simulink model "NN1"  (R2016a)
settings: Solver=VariableStepAuto  StartTime=0.0  StopTime=10.0  RelTol=1e-3
values from neighbouring files (symbols this model uses):
  AaLinear = [0,1,0,0; -(K)/Md,-Rmd/Md,0,A/Md; 0,0,0,1; 0,-A/(L0+Ld),-(1/Cd)/(L0+Ld),-(Re0+Red)/(L0+Ld)]    [NeuroControl_loudspeaker.m]    (also in NeuroControl_loudspeaker2.m; NeuroControl_loudspeaker_LinearPlusNN.m; NeuroControl_loudspeaker_MoreLikeMachineLearning.m; NeuroControl_loudspeaker_MoreLikeMachineLearning_deep.m)
  Anlr = zeros(4,4)    [NeuroControl_loudspeaker.m]    (also in NeuroControl_loudspeaker2.m; NeuroControl_loudspeaker_LinearPlusNN.m; NeuroControl_loudspeaker_MoreLikeMachineLearning.m; NeuroControl_loudspeaker_MoreLikeMachineLearning_deep.m)
  Anlr2 = zeros(4,4)    [NeuroControl_loudspeaker.m]    (also in NeuroControl_loudspeaker2.m; NeuroControl_loudspeaker_LinearPlusNN.m; NeuroControl_loudspeaker_MoreLikeMachineLearning.m; NeuroControl_loudspeaker_MoreLikeMachineLearning_deep.m)
  Anlr3 = zeros(4,4)    [NeuroControl_loudspeaker.m]    (also in NeuroControl_loudspeaker2.m; NeuroControl_loudspeaker_LinearPlusNN.m; NeuroControl_loudspeaker_MoreLikeMachineLearning.m; NeuroControl_loudspeaker_MoreLikeMachineLearning_deep.m)
  Atemp = A    (= 5.62)    [NeuroControl_loudspeaker.m]    (also in NeuroControl_loudspeaker2.m; NeuroControl_loudspeaker_LinearPlusNN.m; NeuroControl_loudspeaker_MoreLikeMachineLearning.m; NeuroControl_loudspeaker_MoreLikeMachineLearning_deep.m)
  Ba = [0,0,0,1/(L0+Ld)]'    [NeuroControl_loudspeaker.m]    (also in NeuroControl_loudspeaker2.m; NeuroControl_loudspeaker_LinearPlusNN.m; NeuroControl_loudspeaker_MoreLikeMachineLearning.m; NeuroControl_loudspeaker_MoreLikeMachineLearning_deep.m)
  K = Kd    (= 4538)    [NeuroControl_loudspeaker.m]    (also in NeuroControl_loudspeaker2.m; NeuroControl_loudspeaker_LinearPlusNN.m; NeuroControl_loudspeaker_MoreLikeMachineLearning.m; NeuroControl_loudspeaker_MoreLikeMachineLearning_deep.m)
  noise = 0    [NeuroControl_loudspeaker.m]    (also in NeuroControl_loudspeaker2.m; NeuroControl_loudspeaker_LinearPlusNN.m; NeuroControl_loudspeaker_MoreLikeMachineLearning.m; NeuroControl_loudspeaker_MoreLikeMachineLearning_deep.m)
  plantInputGainCompensationFb = 1/1.15    (= 0.869565217391)    [NeuroControl_loudspeaker.m]    (also in NeuroControl_loudspeaker2.m; NeuroControl_loudspeaker_LinearPlusNN.m; NeuroControl_loudspeaker_MoreLikeMachineLearning.m; NeuroControl_loudspeaker_MoreLikeMachineLearning_deep.m)
  Rmd = 2.34    [NeuroControl_loudspeaker.m]    (also in NeuroControl_loudspeaker2.m; NeuroControl_loudspeaker_LinearPlusNN.m; NeuroControl_loudspeaker_MoreLikeMachineLearning.m; NeuroControl_loudspeaker_MoreLikeMachineLearning_deep.m)
settings Model: Creator=kadowaki  LastModifiedBy=kadowaki

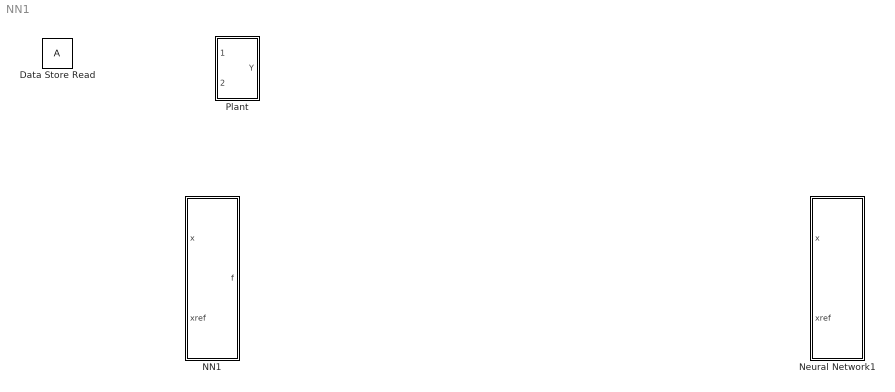
== system NN1 ==
  Data Store Read : DataStoreRead
  NN1 : MATLAB Function  TreatAsAtomicUnit=on
      settings: MinAlgLoopOccurrences=on
  Neural Network1 : MATLAB Function  TreatAsAtomicUnit=on
      settings: MinAlgLoopOccurrences=on
  Plant : Subsystem

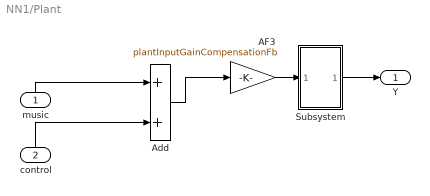
== system NN1/Plant ==
  music : Inport
  control : Inport  Port=2
  AF3 : Gain  Gain=plantInputGainCompensationFb
  Add : Sum
  Subsystem : Subsystem  TreatAsAtomicUnit=on
      settings: MinAlgLoopOccurrences=on
  Y : Outport
  wires:
  Subsystem/1(Out1) -> Y/1
  AF3/1 -> Subsystem/1(In2)
  music/1 -> Add/1
  control/1 -> Add/2
  Add/1 -> AF3/1

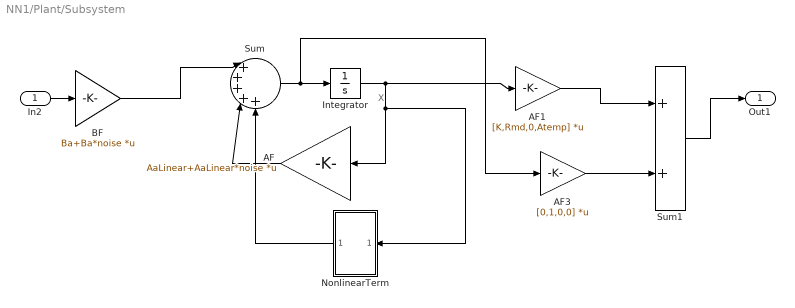
== system NN1/Plant/Subsystem ==
  note: X
  In2 : Inport
  AF : Gain  Gain=AaLinear+AaLinear*noise  Multiplication=Matrix(K*u)
  AF1 : Gain  Gain=[K,Rmd,0,Atemp]  Multiplication=Matrix(K*u)
  AF3 : Gain  Gain=[0,1,0,0]  Multiplication=Matrix(K*u)
  BF : Gain  Gain=Ba+Ba*noise  Multiplication=Matrix(K*u)
  Integrator : Integrator
  NonlinearTerm : Subsystem
  Sum : Sum  Inputs=|+++++
  Sum1 : Sum
  Out1 : Outport
  wires:
  BF/1 -> Sum/1
  Sum/1 -> Integrator/1, AF3/1
  Integrator/1 -> AF/1, NonlinearTerm/1(In1), AF1/1
  AF/1 -> Sum/4
  NonlinearTerm/1(Out2) -> Sum/5
  In2/1 -> BF/1
  AF1/1 -> Sum1/1
  Sum1/1 -> Out1/1
  AF3/1 -> Sum1/2

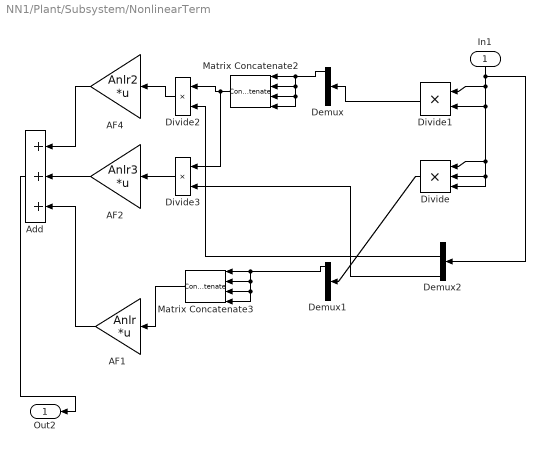
== system NN1/Plant/Subsystem/NonlinearTerm ==
  In1 : Inport
  AF1 : Gain  Gain=Anlr  Multiplication=Matrix(K*u)
  AF2 : Gain  Gain=Anlr3  Multiplication=Matrix(K*u)
  AF4 : Gain  Gain=Anlr2  Multiplication=Matrix(K*u)
  Add : Sum  Inputs=+++
  Demux : Demux  Outputs=[1,1,1,1]
  Demux1 : Demux  Outputs=[1,1,1,1]
  Demux2 : Demux  Outputs=[1,1,1,1]
  Divide : Product  Inputs=***
  Divide1 : Product  Inputs=**
  Divide2 : Product  Inputs=**
  Divide3 : Product  Inputs=**
  Matrix Concatenate2 : Concatenate  NumInputs=4
  Matrix Concatenate3 : Concatenate  NumInputs=4
  Out2 : Outport
  wires:
  Matrix Concatenate3/1 -> AF1/1
  Divide/1 -> Demux1/1
  In1/1 -> Demux2/1, Divide1/2, Divide/2, Divide/3, Divide/1, Divide1/1
  Demux/1 -> Matrix Concatenate2/1, Matrix Concatenate2/2, Matrix Concatenate2/3, Matrix Concatenate2/4
  Demux1/1 -> Matrix Concatenate3/1, Matrix Concatenate3/2, Matrix Concatenate3/3, Matrix Concatenate3/4
  AF2/1 -> Add/2
  AF4/1 -> Add/1
  AF1/1 -> Add/3
  Add/1 -> Out2/1
  Matrix Concatenate2/1 -> Divide2/1, Divide3/1
  Demux2/2 -> Divide2/2
  Divide2/1 -> AF4/1
  Divide3/1 -> AF2/1
  Demux2/4 -> Divide3/2
  Divide1/1 -> Demux/1

== matlab function NN1/Neural Network1 ==
  data: x input; xref input; yOld data_store_memory; duOld data_store_memory
function fcn(x,xref)
%% cost関数をatctual plantの出力YとYrefの差の二乗和の形に書き換える。それにともなってsigKとかも変わる
%%%%%%%%%%%%%%%%%%%%%%%%%%%%%%%%%%%%%%%%%%%%%%%%%%%%%%%%%%%%%%%%%%%%%%%%%%%%%%%%%%%%%%%%%%%%%%%%%%%%%%%%%%%%
%%

%#codegen
%配列は縦で入れる
%PRMLの5.3.2
%隠れ層はtanh,出力層は線形の活性化関数
% Input:
%   x: state vector of a plant
%   xref: reference state vector
%   h: 隠れ層のニューロン数
% Ouput:
%   du: input to compensate plant nonlinearity
%   mse: mean square error
%12input-1outputのニューラルネット
%フィードバックの機構いる？ニューラルネットだけではだめなのか。
%実装に際しては，1サンプル中にニューラルネットの計算が終わるのかという問題はある。

%過去のy保存用のグローバル変数定義
global yOld
global duOld

if isempty(yOld) == 1
    duOld = 0;
    yOld = 0;
end

%隠れ層のレイヤー数
h = 12;
%各レイヤーのユニット数
%h = [size(x,1)+1;h(:)+1;size(xref,1)];
h = [size(x,1)+1;h(:)+1;1];
%レイヤー数
L = numel(h);
W = cell(L-1);
for l = 1:L-1
    W{l} = randn(h(l),h(l+1));
end
du = cell(L);
du{1} = [1;x];
%eta = 1/size(x,2);
eta = 0.01;
maxiter = 4000;
mse = zeros(1,maxiter);
mse(1) = 1;
% %描画準備
% figure(1)
% plot(xref)
% hold on
%iteration variable
iter = 1;
%while mse(iter) > 0.0005
    iter = iter + 1;
    %forward
    %中間層出力
    l = 2;
    
    %活性化関数定義
    du{l} = tanh(W{l-1}'*du{l-1});
    
    %出力層出力
    l = 3;
    du{l} = W{l-1}'*du{l-1};
    
    %ヤコビアンを求める
    deltaU = du{3} - duOld;
    deltaY = y - yOld;
    if deltaU*deltaY < 0
        jacobi = -1;
    elseif deltaU*deltaY == 0
        jacobi = 0;
    else 
        jacobi = 1;
    end
    
    %出力層ユニットに対するsigmaK
    sigK = (y - yref)*jacobi;
    %     backward
    E = y - yref;
    mse(iter) = mean(dot(E(:),E(:)));
    l = 2;
    %         df = (1-Y{l+1}.^2);
    %         dG = df.*E;
    %         dW = Y{l}*dG';
    
    sigJ = (1-du{l}.^2).*(W{l}*sigK);
    
    W{1} = W{1}-eta*(sigJ*du{1}')';
    W{2} = W{2}-eta*(sigK*du{2}')';
    
    %     if mod(iter,10) == 0
    %         figure(1)
    %         plot(Y{L})
    %     end
%     %成長の描画
%     figure(1)
%     ylim([min(xref)*1.2, max(xref)*1.2])
%     plot(du{L})
%     pause(.1)
%end
mse = mse(1:iter);
%model.W = W;
duOut = du{3};
duOld = duOut;
yOld = y;
%disp(['iteration number:',num2str(iter)])

== matlab function NN1/NN1 ==
  data: x input; f output; xref input; yOld data_store_memory; duOld data_store_memory
function f  = fcn(x,xref)
%% cost関数をatctual plantの出力YとYrefの差の二乗和の形に書き換える。それにともなってsigKとかも変わる
%%%%%%%%%%%%%%%%%%%%%%%%%%%%%%%%%%%%%%%%%%%%%%%%%%%%%%%%%%%%%%%%%%%%%%%%%%%%%%%%%%%%%%%%%%%%%%%%%%%%%%%%%%%%
%%

%#codegen
%配列は縦で入れる
%PRMLの5.3.2
%隠れ層はtanh,出力層は線形の活性化関数
% Input:
%   x: state vector of a plant
%   xref: reference state vector
%   h: 隠れ層のニューロン数
% Ouput:
%   du: input to compensate plant nonlinearity
%   mse: mean square error
%12input-1outputのニューラルネット
%フィードバックの機構いる？ニューラルネットだけではだめなのか。
%実装に際しては，1サンプル中にニューラルネットの計算が終わるのかという問題はある。

%過去のy保存用のグローバル変数定義
global yOld
global duOld

if isempty(yOld) == 1
    duOld = 0;
    yOld = 0;
end

%隠れ層のレイヤー数
h = 12;
%各レイヤーのユニット数
%h = [size(x,1)+1;h(:)+1;size(xref,1)];
h = [size(x,1)+1;h(:)+1;1];
%レイヤー数
L = numel(h);
W = cell(L-1);
for l = 1:L-1
    W{l} = randn(h(l),h(l+1));
end
du = cell(L);
du{1} = [1;x];
%eta = 1/size(x,2);
eta = 0.01;
maxiter = 4000;
mse = zeros(1,maxiter);
mse(1) = 1;
% %描画準備
% figure(1)
% plot(xref)
% hold on
%iteration variable
iter = 1;
%while mse(iter) > 0.0005
    iter = iter + 1;
    %forward
    %中間層出力
    l = 2;
    
    %活性化関数定義
    du{l} = tanh(W{l-1}'*du{l-1});
    
    %出力層出力
    l = 3;
    du{l} = W{l-1}'*du{l-1};
    
    %ヤコビアンを求める
    deltaU = du{3} - duOld;
    deltaY = y - yOld;
    if deltaU*deltaY < 0
        jacobi = -1;
    elseif deltaU*deltaY == 0
        jacobi = 0;
    else 
        jacobi = 1;
    end
    
    %出力層ユニットに対するsigmaK
    sigK = (y - yref)*jacobi;
    %     backward
    E = y - yref;
    mse(iter) = mean(dot(E(:),E(:)));
    l = 2;
    %         df = (1-Y{l+1}.^2);
    %         dG = df.*E;
    %         dW = Y{l}*dG';
    
    sigJ = (1-du{l}.^2).*(W{l}*sigK);
    
    W{1} = W{1}-eta*(sigJ*du{1}')';
    W{2} = W{2}-eta*(sigK*du{2}')';
    
    %     if mod(iter,10) == 0
    %         figure(1)
    %         plot(Y{L})
    %     end
%     %成長の描画
%     figure(1)
%     ylim([min(xref)*1.2, max(xref)*1.2])
%     plot(du{L})
%     pause(.1)
%end
mse = mse(1:iter);
%model.W = W;
duOut = du{3};
duOld = duOut;
yOld = y;
%disp(['iteration number:',num2str(iter)])
